simulink model "piddeneme"  (R2022b)
settings: Solver=VariableStepAuto  StartTime=0.0  StopTime=100  RelTol=1e-3
settings Model: Creator=Fatih  LastModifiedBy=Fatih

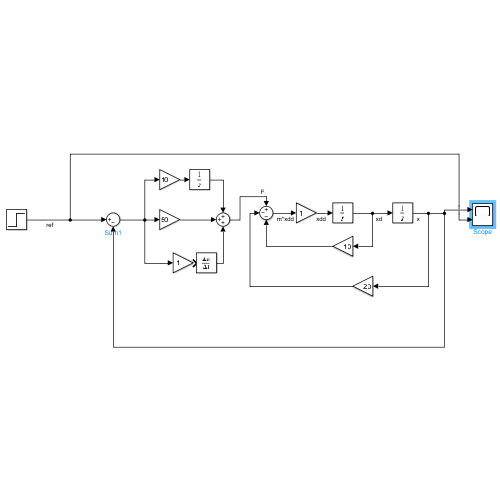
[thumbnail: Simulink's stored preview of the top-level diagram]
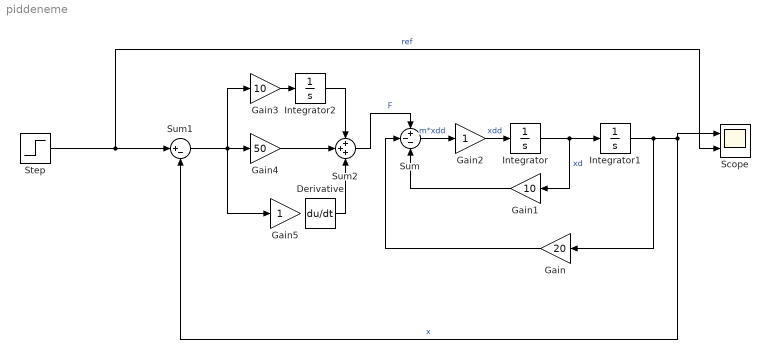
== system piddeneme ==
  Derivative : Derivative
  Gain : Gain  Gain=20
  Gain1 : Gain  Gain=10
  Gain2 : Gain
  Gain3 : Gain  Gain=10
  Gain4 : Gain  Gain=50
  Gain5 : Gain
  Integrator : Integrator
  Integrator1 : Integrator
  Integrator2 : Integrator
  Scope : Scope  NumInputPorts=2
  Step : Step  SampleTime=0
  Sum : Sum  Inputs=+--
  Sum1 : Sum  Inputs=|+-
  Sum2 : Sum  Inputs=+++
  wires:
  Integrator/1 -> Gain1/1, Integrator1/1  "xd"
  Integrator1/1 -> Gain/1, Sum1/2, Scope/1  "x"
  Gain/1 -> Sum/2
  Gain1/1 -> Sum/3
  Sum2/1 -> Sum/1  "F"
  Sum/1 -> Gain2/1  "m*xdd"
  Gain2/1 -> Integrator/1  "xdd"
  Step/1 -> Scope/2, Sum1/1  "ref"
  Sum1/1 -> Gain3/1, Gain5/1, Gain4/1
  Gain3/1 -> Integrator2/1
  Integrator2/1 -> Sum2/1
  Gain4/1 -> Sum2/2
  Derivative/1 -> Sum2/3
